simulink model "pasp_16ip_16ch"  (Simulink 6.2)
settings: Solver=ode45  StartTime=0.0  StopTime=30000  RelTol=1e-3
undefined symbols (not defined in the file or in its folder): iBOB
libraries: xbsIndex_r3 x1479, casper_library x149, xps_library x58
(part 3 of 11)

== system pasp_16ip_16ch/pasp/reorder ==
  sync : Inport  Port=1  LatchInput=off
  en : Inport  Port=2  LatchInput=off
  din0 : Inport  Port=3  LatchInput=off
  din1 : Inport  Port=4  LatchInput=off
  Counter : xbsIndex_r3/Counter  cnt_type=Count Limited  n_bits=6  bin_pt=0  arith_type=Unsigned  start_count=0  cnt_to=63  cnt_by_val=1  operation=Up  explicit_period=off  period=1  load_pin=off  rst=on  en=on  dbl_ovrd=off  show_param=off  use_rpm=on  gen_core=off
      settings: xl_area=[0, 0, 0, 0, 0, 0, 0]
  Mux : xbsIndex_r3/Mux  inputs=4  precision=Full  arith_type="Signed  (2's comp)"  n_bits=8  bin_pt=2  quantization=Truncate  overflow=Wrap  latency=1  explicit_period=off  period=1  en=off  dbl_ovrd=off  show_param=off  mux_type=off  use_rpm=off  gen_core=off
      settings: xl_area=[0, 0, 0, 0, 0, 0, 0]
  Slice1 : xbsIndex_r3/Slice  mode=Upper Bit Location + Width  nbits=2  bit1=0  base1=MSB of Input  bit0=0  base0=LSB of Input  boolean_output=off  explicit_period=off  period=1  dbl_ovrd=off
  Slice2 : xbsIndex_r3/Slice  mode=Lower Bit Location + Width  nbits=4  bit1=0  base1=MSB of Input  bit0=0  base0=LSB of Input  boolean_output=off  explicit_period=off  period=1  dbl_ovrd=off
  bram0 : xbsIndex_r3/Single Port RAM  depth=16  initVector=sin(pi*(0:15)/16)  write_mode=Read Before Write  latency=2  init_zero=on  explicit_period=off  period=1  rst=off  init_reg=0  en=off  dbl_ovrd=off  show_param=off  distributed_mem=off  use_rpm=off  gen_core=off
      settings: xl_area=[0, 0, 0, 0, 0, 0, 0]
  bram1 : xbsIndex_r3/Single Port RAM  depth=16  initVector=sin(pi*(0:15)/16)  write_mode=Read Before Write  latency=2  init_zero=on  explicit_period=off  period=1  rst=off  init_reg=0  en=off  dbl_ovrd=off  show_param=off  distributed_mem=off  use_rpm=off  gen_core=off
      settings: xl_area=[0, 0, 0, 0, 0, 0, 0]
  delay_d0 : xbsIndex_r3/Delay  latency=3  reg_retiming=off  explicit_period=off  period=1  en=off  accept_only_valid=off  init_zero=on  dbl_ovrd=off  show_param=off
      settings: xl_area=[0, 0, 0, 0, 0, 0, 0]
  delay_din0 : xbsIndex_r3/Delay  latency=4  reg_retiming=off  explicit_period=off  period=1  en=off  accept_only_valid=off  init_zero=on  dbl_ovrd=off  show_param=off
      settings: xl_area=[0, 0, 0, 0, 0, 0, 0]
  delay_din1 : xbsIndex_r3/Delay  latency=4  reg_retiming=off  explicit_period=off  period=1  en=off  accept_only_valid=off  init_zero=on  dbl_ovrd=off  show_param=off
      settings: xl_area=[0, 0, 0, 0, 0, 0, 0]
  delay_map1 : xbsIndex_r3/Delay  latency=2*map_latency  reg_retiming=off  explicit_period=off  period=1  en=off  accept_only_valid=off  init_zero=on  dbl_ovrd=off  show_param=off
      settings: xl_area=[0, 0, 0, 0, 0, 0, 0]
  delay_map2 : xbsIndex_r3/Delay  latency=1*map_latency  reg_retiming=off  explicit_period=off  period=1  en=off  accept_only_valid=off  init_zero=on  dbl_ovrd=off  show_param=off
      settings: xl_area=[0, 0, 0, 0, 0, 0, 0]
  delay_map3 : xbsIndex_r3/Delay  latency=0*map_latency  reg_retiming=off  explicit_period=off  period=1  en=off  accept_only_valid=off  init_zero=on  dbl_ovrd=off  show_param=off
      settings: xl_area=[0, 0, 0, 0, 0, 0, 0]
  delay_sel : xbsIndex_r3/Delay  latency=3  reg_retiming=off  explicit_period=off  period=1  en=off  accept_only_valid=off  init_zero=on  dbl_ovrd=off  show_param=off
      settings: xl_area=[0, 0, 0, 0, 0, 0, 0]
  delay_valid : xbsIndex_r3/Delay  latency=3  reg_retiming=off  explicit_period=off  period=1  en=off  accept_only_valid=off  init_zero=on  dbl_ovrd=off  show_param=off
      settings: xl_area=[0, 0, 0, 0, 0, 0, 0]
  delay_we : xbsIndex_r3/Delay  latency=3  reg_retiming=off  explicit_period=off  period=1  en=off  accept_only_valid=off  init_zero=on  dbl_ovrd=off  show_param=off
      settings: xl_area=[0, 0, 0, 0, 0, 0, 0]
  map1 : xbsIndex_r3/ROM  depth=16  initVector=[0 8 1 9 2 10 3 11 4 12 5 13 6 14 7 15]  arith_type=Unsigned  n_bits=4  bin_pt=0  latency=1  init_zero=on  explicit_period=off  period=1  rst=off  init_reg=0  en=off  dbl_ovrd=off  show_param=off  distributed_mem=on  use_rpm=off  gen_core=off
      settings: xl_area=[0, 0, 0, 0, 0, 0, 0]
  map2 : xbsIndex_r3/ROM  depth=16  initVector=[0 8 1 9 2 10 3 11 4 12 5 13 6 14 7 15]  arith_type=Unsigned  n_bits=4  bin_pt=0  latency=1  init_zero=on  explicit_period=off  period=1  rst=off  init_reg=0  en=off  dbl_ovrd=off  show_param=off  distributed_mem=on  use_rpm=off  gen_core=off
      settings: xl_area=[0, 0, 0, 0, 0, 0, 0]
  map3 : xbsIndex_r3/ROM  depth=16  initVector=[0 8 1 9 2 10 3 11 4 12 5 13 6 14 7 15]  arith_type=Unsigned  n_bits=4  bin_pt=0  latency=1  init_zero=on  explicit_period=off  period=1  rst=off  init_reg=0  en=off  dbl_ovrd=off  show_param=off  distributed_mem=on  use_rpm=off  gen_core=off
      settings: xl_area=[0, 0, 0, 0, 0, 0, 0]
  post_sync_delay : xbsIndex_r3/Delay  latency=3  reg_retiming=off  explicit_period=off  period=1  en=off  accept_only_valid=off  init_zero=on  dbl_ovrd=off  show_param=off
      settings: xl_area=[0, 0, 0, 0, 0, 0, 0]
  pre_sync_delay : xbsIndex_r3/Delay  latency=3  reg_retiming=off  explicit_period=off  period=1  en=off  accept_only_valid=off  init_zero=on  dbl_ovrd=off  show_param=off
      settings: xl_area=[0, 0, 0, 0, 0, 0, 0]
  sync_delay_en : casper_library/Delays/sync_delay_en  DelayLen=16
      link override Constant: equ=P=C
      link override Constant1: equ=P=C
      link override Constant2: equ=P=C
      link override Constant3: equ=P=C
  sync_out : Outport
  valid : Outport  Port=2
  dout0 : Outport  Port=3
  dout1 : Outport  Port=4
  wires:
  sync/1 -> Counter/1, pre_sync_delay/1
  en/1 -> Counter/2, sync_delay_en/2, delay_we/1
  Counter/1 -> Slice1/1, Slice2/1
  Slice1/1 -> delay_sel/1
  delay_sel/1 -> Mux/1
  Slice2/1 -> delay_d0/1, map1/1
  delay_d0/1 -> Mux/2
  pre_sync_delay/1 -> sync_delay_en/1
  sync_delay_en/1 -> post_sync_delay/1
  post_sync_delay/1 -> sync_out/1
  delay_we/1 -> delay_valid/1, bram0/3, bram1/3
  delay_valid/1 -> valid/1
  Mux/1 -> bram0/1, bram1/1
  din0/1 -> delay_din0/1
  delay_din0/1 -> bram0/2
  bram0/1 -> dout0/1
  din1/1 -> delay_din1/1
  delay_din1/1 -> bram1/2
  bram1/1 -> dout1/1
  map1/1 -> delay_map1/1, map2/1
  delay_map1/1 -> Mux/3
  map2/1 -> delay_map2/1, map3/1
  delay_map2/1 -> Mux/4
  map3/1 -> delay_map3/1
  delay_map3/1 -> Mux/5

== system pasp_16ip_16ch/pasp/scale1 ==
  note: Unsigned, 18-bits, b.p. at 12
  note: Output complex signed R/I 18-bits, b.p. at 17
  note: Input complex signed R/I 18-bits, b.p. at 17
  coeff : Inport  Orientation=down  Port=1  LatchInput=off
  data_in : Inport  Port=2  LatchInput=off
  c_to_ri : casper_library/Misc/c_to_ri  n_bits=18  bin_pt=17
      settings: AttributesFormatString=18_17 r/i
  mult_coeff_fft_imag : xbsIndex_r3/Mult  precision=User Defined  arith_type="Signed  (2's comp)"  n_bits=18  bin_pt=17  quantization=Truncate  overflow=Saturate  latency=6  explicit_period=off  period=1  en=off  dbl_ovrd=off  show_param=on  mult_type=Parallel  oversample=2  use_embedded=on  pipeline=on  use_rpm=on  placement_style=Rectangular Shape  gen_core=off
      settings: xl_area=[0, 0, 0, 0, 0, 0, 0]
  mult_coeff_fft_real : xbsIndex_r3/Mult  precision=User Defined  arith_type="Signed  (2's comp)"  n_bits=18  bin_pt=17  quantization=Truncate  overflow=Saturate  latency=6  explicit_period=off  period=1  en=off  dbl_ovrd=off  show_param=on  mult_type=Parallel  oversample=2  use_embedded=on  pipeline=on  use_rpm=on  placement_style=Rectangular Shape  gen_core=off
      settings: xl_area=[0, 0, 0, 0, 0, 0, 0]
  ri_to_c : casper_library/Misc/ri_to_c
  data_out : Outport
  wires:
  c_to_ri/1 -> mult_coeff_fft_real/2
  c_to_ri/2 -> mult_coeff_fft_imag/2
  mult_coeff_fft_real/1 -> ri_to_c/1
  mult_coeff_fft_imag/1 -> ri_to_c/2
  coeff/1 -> mult_coeff_fft_real/1, mult_coeff_fft_imag/1
  ri_to_c/1 -> data_out/1
  data_in/1 -> c_to_ri/1

== system pasp_16ip_16ch/pasp/scale2 ==
  note: Input complex signed R/I 18-bits, b.p. at 17
  note: Output complex signed R/I 18-bits, b.p. at 17
  note: Unsigned, 18-bits, b.p. at 12
  coeff : Inport  Orientation=down  Port=1  LatchInput=off
  data_in : Inport  Port=2  LatchInput=off
  c_to_ri : casper_library/Misc/c_to_ri  n_bits=18  bin_pt=17
      settings: AttributesFormatString=18_17 r/i
  mult_coeff_fft_imag : xbsIndex_r3/Mult  precision=User Defined  arith_type="Signed  (2's comp)"  n_bits=18  bin_pt=17  quantization=Truncate  overflow=Saturate  latency=6  explicit_period=off  period=1  en=off  dbl_ovrd=off  show_param=on  mult_type=Parallel  oversample=2  use_embedded=on  pipeline=on  use_rpm=on  placement_style=Rectangular Shape  gen_core=off
      settings: xl_area=[0, 0, 0, 0, 0, 0, 0]
  mult_coeff_fft_real : xbsIndex_r3/Mult  precision=User Defined  arith_type="Signed  (2's comp)"  n_bits=18  bin_pt=17  quantization=Truncate  overflow=Saturate  latency=6  explicit_period=off  period=1  en=off  dbl_ovrd=off  show_param=on  mult_type=Parallel  oversample=2  use_embedded=on  pipeline=on  use_rpm=on  placement_style=Rectangular Shape  gen_core=off
      settings: xl_area=[0, 0, 0, 0, 0, 0, 0]
  ri_to_c : casper_library/Misc/ri_to_c
  data_out : Outport
  wires:
  data_in/1 -> c_to_ri/1
  ri_to_c/1 -> data_out/1
  coeff/1 -> mult_coeff_fft_imag/1, mult_coeff_fft_real/1
  mult_coeff_fft_imag/1 -> ri_to_c/2
  mult_coeff_fft_real/1 -> ri_to_c/1
  c_to_ri/2 -> mult_coeff_fft_imag/2
  c_to_ri/1 -> mult_coeff_fft_real/2

== system pasp_16ip_16ch/pasp/scale3 ==
  note: Unsigned, 18-bits, b.p. at 12
  note: Output complex signed R/I 18-bits, b.p. at 17
  note: Input complex signed R/I 18-bits, b.p. at 17
  coeff : Inport  Orientation=down  Port=1  LatchInput=off
  data_in : Inport  Port=2  LatchInput=off
  c_to_ri : casper_library/Misc/c_to_ri  n_bits=18  bin_pt=17
      settings: AttributesFormatString=18_17 r/i
  mult_coeff_fft_imag : xbsIndex_r3/Mult  precision=User Defined  arith_type="Signed  (2's comp)"  n_bits=18  bin_pt=17  quantization=Truncate  overflow=Saturate  latency=6  explicit_period=off  period=1  en=off  dbl_ovrd=off  show_param=on  mult_type=Parallel  oversample=2  use_embedded=on  pipeline=on  use_rpm=on  placement_style=Rectangular Shape  gen_core=off
      settings: xl_area=[0, 0, 0, 0, 0, 0, 0]
  mult_coeff_fft_real : xbsIndex_r3/Mult  precision=User Defined  arith_type="Signed  (2's comp)"  n_bits=18  bin_pt=17  quantization=Truncate  overflow=Saturate  latency=6  explicit_period=off  period=1  en=off  dbl_ovrd=off  show_param=on  mult_type=Parallel  oversample=2  use_embedded=on  pipeline=on  use_rpm=on  placement_style=Rectangular Shape  gen_core=off
      settings: xl_area=[0, 0, 0, 0, 0, 0, 0]
  ri_to_c : casper_library/Misc/ri_to_c
  data_out : Outport
  wires:
  c_to_ri/1 -> mult_coeff_fft_real/2
  c_to_ri/2 -> mult_coeff_fft_imag/2
  mult_coeff_fft_real/1 -> ri_to_c/1
  mult_coeff_fft_imag/1 -> ri_to_c/2
  coeff/1 -> mult_coeff_fft_real/1, mult_coeff_fft_imag/1
  ri_to_c/1 -> data_out/1
  data_in/1 -> c_to_ri/1

== system pasp_16ip_16ch/pasp/scale4 ==
  note: Input complex signed R/I 18-bits, b.p. at 17
  note: Output complex signed R/I 18-bits, b.p. at 17
  note: Unsigned, 18-bits, b.p. at 12
  coeff : Inport  Orientation=down  Port=1  LatchInput=off
  data_in : Inport  Port=2  LatchInput=off
  c_to_ri : casper_library/Misc/c_to_ri  n_bits=18  bin_pt=17
      settings: AttributesFormatString=18_17 r/i
  mult_coeff_fft_imag : xbsIndex_r3/Mult  precision=User Defined  arith_type="Signed  (2's comp)"  n_bits=18  bin_pt=17  quantization=Truncate  overflow=Saturate  latency=6  explicit_period=off  period=1  en=off  dbl_ovrd=off  show_param=on  mult_type=Parallel  oversample=2  use_embedded=on  pipeline=on  use_rpm=on  placement_style=Rectangular Shape  gen_core=off
      settings: xl_area=[0, 0, 0, 0, 0, 0, 0]
  mult_coeff_fft_real : xbsIndex_r3/Mult  precision=User Defined  arith_type="Signed  (2's comp)"  n_bits=18  bin_pt=17  quantization=Truncate  overflow=Saturate  latency=6  explicit_period=off  period=1  en=off  dbl_ovrd=off  show_param=on  mult_type=Parallel  oversample=2  use_embedded=on  pipeline=on  use_rpm=on  placement_style=Rectangular Shape  gen_core=off
      settings: xl_area=[0, 0, 0, 0, 0, 0, 0]
  ri_to_c : casper_library/Misc/ri_to_c
  data_out : Outport
  wires:
  data_in/1 -> c_to_ri/1
  ri_to_c/1 -> data_out/1
  coeff/1 -> mult_coeff_fft_imag/1, mult_coeff_fft_real/1
  mult_coeff_fft_imag/1 -> ri_to_c/2
  mult_coeff_fft_real/1 -> ri_to_c/1
  c_to_ri/2 -> mult_coeff_fft_imag/2
  c_to_ri/1 -> mult_coeff_fft_real/2

== system pasp_16ip_16ch/pasp/scope_output1 ==
  rst : Inport  Port=1  LatchInput=off
  en : Inport  Port=2  LatchInput=off
  data_in : Inport  Port=3  LatchInput=off
  bram : xps_library/Shared BRAM  Tag=xps:bram  arith_type="Signed  (2's comp)"  addr_width=11  data_width=32  data_bin_pt=17  init_vals=[1:2^11]  sample_rate=1
  freeze_cntr : casper_library/Misc/freeze_cntr  CounterBits=11
  wires:
  freeze_cntr/1 -> bram/1
  freeze_cntr/2 -> bram/3
  en/1 -> freeze_cntr/1
  data_in/1 -> bram/2
  rst/1 -> freeze_cntr/2

== system pasp_16ip_16ch/pasp/scope_output2 ==
  rst : Inport  Port=1  LatchInput=off
  en : Inport  Port=2  LatchInput=off
  data_in : Inport  Port=3  LatchInput=off
  bram : xps_library/Shared BRAM  Tag=xps:bram  arith_type="Signed  (2's comp)"  addr_width=11  data_width=32  data_bin_pt=17  init_vals=[1:2^11]  sample_rate=1
  freeze_cntr : casper_library/Misc/freeze_cntr  CounterBits=11
  wires:
  freeze_cntr/1 -> bram/1
  freeze_cntr/2 -> bram/3
  en/1 -> freeze_cntr/1
  data_in/1 -> bram/2
  rst/1 -> freeze_cntr/2

== system pasp_16ip_16ch/pasp/scope_output3 ==
  rst : Inport  Port=1  LatchInput=off
  en : Inport  Port=2  LatchInput=off
  data_in : Inport  Port=3  LatchInput=off
  bram : xps_library/Shared BRAM  Tag=xps:bram  arith_type="Signed  (2's comp)"  addr_width=11  data_width=32  data_bin_pt=17  init_vals=[1:2^11]  sample_rate=1
  freeze_cntr : casper_library/Misc/freeze_cntr  CounterBits=11
  wires:
  rst/1 -> freeze_cntr/2
  data_in/1 -> bram/2
  en/1 -> freeze_cntr/1
  freeze_cntr/2 -> bram/3
  freeze_cntr/1 -> bram/1

== system pasp_16ip_16ch/pasp/scope_output4 ==
  rst : Inport  Port=1  LatchInput=off
  en : Inport  Port=2  LatchInput=off
  data_in : Inport  Port=3  LatchInput=off
  bram : xps_library/Shared BRAM  Tag=xps:bram  arith_type="Signed  (2's comp)"  addr_width=11  data_width=32  data_bin_pt=17  init_vals=[1:2^11]  sample_rate=1
  freeze_cntr : casper_library/Misc/freeze_cntr  CounterBits=11
  wires:
  freeze_cntr/1 -> bram/1
  freeze_cntr/2 -> bram/3
  en/1 -> freeze_cntr/1
  data_in/1 -> bram/2
  rst/1 -> freeze_cntr/2

== system pasp_16ip_16ch/pasp/scope_output5 ==
  rst : Inport  Port=1  LatchInput=off
  en : Inport  Port=2  LatchInput=off
  data_in : Inport  Port=3  LatchInput=off
  bram : xps_library/Shared BRAM  Tag=xps:bram  arith_type="Signed  (2's comp)"  addr_width=11  data_width=32  data_bin_pt=17  init_vals=[1:2^11]  sample_rate=1
  freeze_cntr : casper_library/Misc/freeze_cntr  CounterBits=11
  wires:
  freeze_cntr/1 -> bram/1
  freeze_cntr/2 -> bram/3
  en/1 -> freeze_cntr/1
  data_in/1 -> bram/2
  rst/1 -> freeze_cntr/2

== system pasp_16ip_16ch/pasp/scope_output6 ==
  rst : Inport  Port=1  LatchInput=off
  en : Inport  Port=2  LatchInput=off
  data_in : Inport  Port=3  LatchInput=off
  bram : xps_library/Shared BRAM  Tag=xps:bram  arith_type="Signed  (2's comp)"  addr_width=11  data_width=32  data_bin_pt=17  init_vals=[1:2^11]  sample_rate=1
  freeze_cntr : casper_library/Misc/freeze_cntr  CounterBits=11
  wires:
  freeze_cntr/1 -> bram/1
  freeze_cntr/2 -> bram/3
  en/1 -> freeze_cntr/1
  data_in/1 -> bram/2
  rst/1 -> freeze_cntr/2

== system pasp_16ip_16ch/pasp/scope_output7 ==
  rst : Inport  Port=1  LatchInput=off
  en : Inport  Port=2  LatchInput=off
  data_in : Inport  Port=3  LatchInput=off
  bram : xps_library/Shared BRAM  Tag=xps:bram  arith_type="Signed  (2's comp)"  addr_width=11  data_width=32  data_bin_pt=17  init_vals=[1:2^11]  sample_rate=1
  freeze_cntr : casper_library/Misc/freeze_cntr  CounterBits=11
  wires:
  rst/1 -> freeze_cntr/2
  data_in/1 -> bram/2
  en/1 -> freeze_cntr/1
  freeze_cntr/2 -> bram/3
  freeze_cntr/1 -> bram/1

== system pasp_16ip_16ch/pasp/scope_output8 ==
  rst : Inport  Port=1  LatchInput=off
  en : Inport  Port=2  LatchInput=off
  data_in : Inport  Port=3  LatchInput=off
  bram : xps_library/Shared BRAM  Tag=xps:bram  arith_type="Signed  (2's comp)"  addr_width=11  data_width=32  data_bin_pt=17  init_vals=[1:2^11]  sample_rate=1
  freeze_cntr : casper_library/Misc/freeze_cntr  CounterBits=11
  wires:
  freeze_cntr/1 -> bram/1
  freeze_cntr/2 -> bram/3
  en/1 -> freeze_cntr/1
  data_in/1 -> bram/2
  rst/1 -> freeze_cntr/2

== system pasp_16ip_16ch/pasp/sync_generator ==
  period : Inport  Port=1  LatchInput=off
  reset : Inport  Port=2  LatchInput=off
  Convert : xbsIndex_r3/Convert  arith_type=Boolean  n_bits=8  bin_pt=6  quantization=Truncate  overflow=Wrap  latency=1  explicit_period=off  period=1  dbl_ovrd=off  show_param=off  inserted_by_tool=off  pipeline=off
      settings: xl_area=[0, 0, 0, 0, 0, 0, 0]
  Counter : xbsIndex_r3/Counter  cnt_type=Free Running  n_bits=32  bin_pt=0  arith_type=Unsigned  start_count=1  cnt_to=Inf  cnt_by_val=1  operation=Up  explicit_period=on  period=1  load_pin=off  rst=on  en=off  dbl_ovrd=off  show_param=off  use_rpm=on  gen_core=off
      settings: xl_area=[0, 0, 0, 0, 0, 0, 0]
  Logical : xbsIndex_r3/Logical  logical_function=OR  inputs=2  precision=Full  arith_type=Unsigned  n_bits=8  bin_pt=2  align_bp=on  latency=0  explicit_period=off  period=1  en=off  dbl_ovrd=off  show_param=off
      settings: xl_area=[0, 0, 0, 0, 0, 0, 0]
  Relational : xbsIndex_r3/Relational  mode=a>=b  latency=1  explicit_period=off  period=1  en=off  dbl_ovrd=off  show_param=off
      settings: xl_area=[0, 0, 0, 0, 0, 0, 0]
  cns : xbsIndex_r3/Constant  const=4  equ=P=C  arith_type=Unsigned  n_bits=3  bin_pt=0  opselect=C  inp2=PCIN>>17  opr=+  inp1=P  carry=CIN  iostate=0  explicit_period=off  period=1  dbl_ovrd=off
  period_sub : xbsIndex_r3/AddSub  mode=Subtraction  precision=User Defined  arith_type=Unsigned  n_bits=32  bin_pt=0  quantization=Truncate  overflow=Wrap  latency=0  explicit_period=off  period=1  use_carryin=off  use_carryout=off  en=off  dbl_ovrd=off  show_param=off  use_core=on  pipeline=off  use_rpm=on  gen_core=off
      settings: xl_area=[0, 0, 0, 0, 0, 0, 0]
  posedge : casper_library/Misc/posedge  Tag=Rising Edge Detector
  sync : Outport
  wires:
  Counter/1 -> Relational/1
  Relational/1 -> Convert/1
  Convert/1 -> Logical/2
  Logical/1 -> Counter/1, posedge/1
  reset/1 -> Logical/1
  period/1 -> period_sub/1
  period_sub/1 -> Relational/2
  cns/1 -> period_sub/2
  posedge/1 -> sync/1

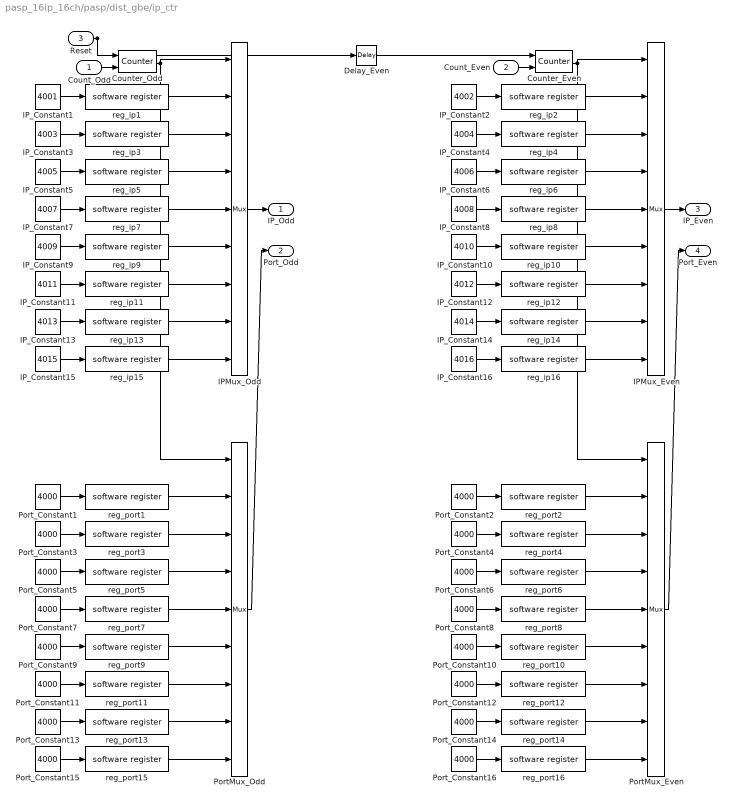
== system pasp_16ip_16ch/pasp/dist_gbe/ip_ctr ==
  Count_Odd : Inport  Port=1  LatchInput=off
  Count_Even : Inport  Port=2  LatchInput=off
  Reset : Inport  Port=3  LatchInput=off
  Counter_Even : xbsIndex_r3/Counter  cnt_type=Free Running  n_bits=3  bin_pt=0  arith_type=Unsigned  start_count=0  cnt_to=Inf  cnt_by_val=1  operation=Up  explicit_period=off  period=1  load_pin=off  rst=on  en=on  dbl_ovrd=off  show_param=off  use_rpm=on  gen_core=off
      settings: xl_area=[0, 0, 0, 0, 0, 0, 0]
  Counter_Odd : xbsIndex_r3/Counter  cnt_type=Free Running  n_bits=3  bin_pt=0  arith_type=Unsigned  start_count=0  cnt_to=Inf  cnt_by_val=1  operation=Up  explicit_period=off  period=1  load_pin=off  rst=on  en=on  dbl_ovrd=off  show_param=off  use_rpm=on  gen_core=off
      settings: xl_area=[0, 0, 0, 0, 0, 0, 0]
  Delay_Even : xbsIndex_r3/Delay  latency=4  reg_retiming=off  explicit_period=off  period=1  en=off  accept_only_valid=off  init_zero=on  dbl_ovrd=off  show_param=off
      settings: xl_area=[0, 0, 0, 0, 0, 0, 0]
  IPMux_Even : xbsIndex_r3/Mux  inputs=8  precision=Full  arith_type="Signed  (2's comp)"  n_bits=8  bin_pt=2  quantization=Truncate  overflow=Wrap  latency=3  explicit_period=off  period=1  en=off  dbl_ovrd=off  show_param=off  mux_type=off  use_rpm=off  gen_core=off
      settings: xl_area=[0, 0, 0, 0, 0, 0, 0]
  IPMux_Odd : xbsIndex_r3/Mux  inputs=8  precision=Full  arith_type="Signed  (2's comp)"  n_bits=8  bin_pt=2  quantization=Truncate  overflow=Wrap  latency=3  explicit_period=off  period=1  en=off  dbl_ovrd=off  show_param=off  mux_type=off  use_rpm=off  gen_core=off
      settings: xl_area=[0, 0, 0, 0, 0, 0, 0]
  IP_Constant1 : Constant  Value=4001
  IP_Constant10 : Constant  Value=4010
  IP_Constant11 : Constant  Value=4011
  IP_Constant12 : Constant  Value=4012
  IP_Constant13 : Constant  Value=4013
  IP_Constant14 : Constant  Value=4014
  IP_Constant15 : Constant  Value=4015
  IP_Constant16 : Constant  Value=4016
  IP_Constant2 : Constant  Value=4002
  IP_Constant3 : Constant  Value=4003
  IP_Constant4 : Constant  Value=4004
  IP_Constant5 : Constant  Value=4005
  IP_Constant6 : Constant  Value=4006
  IP_Constant7 : Constant  Value=4007
  IP_Constant8 : Constant  Value=4008
  IP_Constant9 : Constant  Value=4009
  PortMux_Even : xbsIndex_r3/Mux  inputs=8  precision=Full  arith_type="Signed  (2's comp)"  n_bits=8  bin_pt=2  quantization=Truncate  overflow=Wrap  latency=3  explicit_period=off  period=1  en=off  dbl_ovrd=off  show_param=off  mux_type=off  use_rpm=off  gen_core=off
      settings: xl_area=[0, 0, 0, 0, 0, 0, 0]
  PortMux_Odd : xbsIndex_r3/Mux  inputs=8  precision=Full  arith_type="Signed  (2's comp)"  n_bits=8  bin_pt=2  quantization=Truncate  overflow=Wrap  latency=3  explicit_period=off  period=1  en=off  dbl_ovrd=off  show_param=off  mux_type=off  use_rpm=off  gen_core=off
      settings: xl_area=[0, 0, 0, 0, 0, 0, 0]
  Port_Constant{1..16} (16 alike) : Constant  Value=4000
  reg_ip1 : xps_library/software register  Tag=xps:sw_reg  io_dir=From Processor  arith_type=Unsigned  bitwidth=32  bin_pt=0  sample_period=1  gw_name=pasp_16ip_16ch_pasp_dist_gbe_ip_ctr_reg_ip1_user_data_out
  reg_ip10 : xps_library/software register  Tag=xps:sw_reg  io_dir=From Processor  arith_type=Unsigned  bitwidth=32  bin_pt=0  sample_period=1  gw_name=pasp_16ip_16ch_pasp_dist_gbe_ip_ctr_reg_ip10_user_data_out
  reg_ip11 : xps_library/software register  Tag=xps:sw_reg  io_dir=From Processor  arith_type=Unsigned  bitwidth=32  bin_pt=0  sample_period=1  gw_name=pasp_16ip_16ch_pasp_dist_gbe_ip_ctr_reg_ip11_user_data_out
  reg_ip12 : xps_library/software register  Tag=xps:sw_reg  io_dir=From Processor  arith_type=Unsigned  bitwidth=32  bin_pt=0  sample_period=1  gw_name=pasp_16ip_16ch_pasp_dist_gbe_ip_ctr_reg_ip12_user_data_out
  reg_ip13 : xps_library/software register  Tag=xps:sw_reg  io_dir=From Processor  arith_type=Unsigned  bitwidth=32  bin_pt=0  sample_period=1  gw_name=pasp_16ip_16ch_pasp_dist_gbe_ip_ctr_reg_ip13_user_data_out
  reg_ip14 : xps_library/software register  Tag=xps:sw_reg  io_dir=From Processor  arith_type=Unsigned  bitwidth=32  bin_pt=0  sample_period=1  gw_name=pasp_16ip_16ch_pasp_dist_gbe_ip_ctr_reg_ip14_user_data_out
  reg_ip15 : xps_library/software register  Tag=xps:sw_reg  io_dir=From Processor  arith_type=Unsigned  bitwidth=32  bin_pt=0  sample_period=1  gw_name=pasp_16ip_16ch_pasp_dist_gbe_ip_ctr_reg_ip15_user_data_out
  reg_ip16 : xps_library/software register  Tag=xps:sw_reg  io_dir=From Processor  arith_type=Unsigned  bitwidth=32  bin_pt=0  sample_period=1  gw_name=pasp_16ip_16ch_pasp_dist_gbe_ip_ctr_reg_ip16_user_data_out
  reg_ip2 : xps_library/software register  Tag=xps:sw_reg  io_dir=From Processor  arith_type=Unsigned  bitwidth=32  bin_pt=0  sample_period=1  gw_name=pasp_16ip_16ch_pasp_dist_gbe_ip_ctr_reg_ip2_user_data_out
  reg_ip3 : xps_library/software register  Tag=xps:sw_reg  io_dir=From Processor  arith_type=Unsigned  bitwidth=32  bin_pt=0  sample_period=1  gw_name=pasp_16ip_16ch_pasp_dist_gbe_ip_ctr_reg_ip3_user_data_out
  reg_ip4 : xps_library/software register  Tag=xps:sw_reg  io_dir=From Processor  arith_type=Unsigned  bitwidth=32  bin_pt=0  sample_period=1  gw_name=pasp_16ip_16ch_pasp_dist_gbe_ip_ctr_reg_ip4_user_data_out
  reg_ip5 : xps_library/software register  Tag=xps:sw_reg  io_dir=From Processor  arith_type=Unsigned  bitwidth=32  bin_pt=0  sample_period=1  gw_name=pasp_16ip_16ch_pasp_dist_gbe_ip_ctr_reg_ip5_user_data_out
  reg_ip6 : xps_library/software register  Tag=xps:sw_reg  io_dir=From Processor  arith_type=Unsigned  bitwidth=32  bin_pt=0  sample_period=1  gw_name=pasp_16ip_16ch_pasp_dist_gbe_ip_ctr_reg_ip6_user_data_out
  reg_ip7 : xps_library/software register  Tag=xps:sw_reg  io_dir=From Processor  arith_type=Unsigned  bitwidth=32  bin_pt=0  sample_period=1  gw_name=pasp_16ip_16ch_pasp_dist_gbe_ip_ctr_reg_ip7_user_data_out
  reg_ip8 : xps_library/software register  Tag=xps:sw_reg  io_dir=From Processor  arith_type=Unsigned  bitwidth=32  bin_pt=0  sample_period=1  gw_name=pasp_16ip_16ch_pasp_dist_gbe_ip_ctr_reg_ip8_user_data_out
  reg_ip9 : xps_library/software register  Tag=xps:sw_reg  io_dir=From Processor  arith_type=Unsigned  bitwidth=32  bin_pt=0  sample_period=1  gw_name=pasp_16ip_16ch_pasp_dist_gbe_ip_ctr_reg_ip9_user_data_out
  reg_port1 : xps_library/software register  Tag=xps:sw_reg  io_dir=From Processor  arith_type=Unsigned  bitwidth=32  bin_pt=0  sample_period=1  gw_name=pasp_16ip_16ch_pasp_dist_gbe_ip_ctr_reg_port1_user_data_out
  reg_port10 : xps_library/software register  Tag=xps:sw_reg  io_dir=From Processor  arith_type=Unsigned  bitwidth=32  bin_pt=0  sample_period=1  gw_name=pasp_16ip_16ch_pasp_dist_gbe_ip_ctr_reg_port10_user_data_out
  reg_port11 : xps_library/software register  Tag=xps:sw_reg  io_dir=From Processor  arith_type=Unsigned  bitwidth=32  bin_pt=0  sample_period=1  gw_name=pasp_16ip_16ch_pasp_dist_gbe_ip_ctr_reg_port11_user_data_out
  reg_port12 : xps_library/software register  Tag=xps:sw_reg  io_dir=From Processor  arith_type=Unsigned  bitwidth=32  bin_pt=0  sample_period=1  gw_name=pasp_16ip_16ch_pasp_dist_gbe_ip_ctr_reg_port12_user_data_out
  reg_port13 : xps_library/software register  Tag=xps:sw_reg  io_dir=From Processor  arith_type=Unsigned  bitwidth=32  bin_pt=0  sample_period=1  gw_name=pasp_16ip_16ch_pasp_dist_gbe_ip_ctr_reg_port13_user_data_out
  reg_port14 : xps_library/software register  Tag=xps:sw_reg  io_dir=From Processor  arith_type=Unsigned  bitwidth=32  bin_pt=0  sample_period=1  gw_name=pasp_16ip_16ch_pasp_dist_gbe_ip_ctr_reg_port14_user_data_out
  reg_port15 : xps_library/software register  Tag=xps:sw_reg  io_dir=From Processor  arith_type=Unsigned  bitwidth=32  bin_pt=0  sample_period=1  gw_name=pasp_16ip_16ch_pasp_dist_gbe_ip_ctr_reg_port15_user_data_out
  reg_port16 : xps_library/software register  Tag=xps:sw_reg  io_dir=From Processor  arith_type=Unsigned  bitwidth=32  bin_pt=0  sample_period=1  gw_name=pasp_16ip_16ch_pasp_dist_gbe_ip_ctr_reg_port16_user_data_out
  reg_port2 : xps_library/software register  Tag=xps:sw_reg  io_dir=From Processor  arith_type=Unsigned  bitwidth=32  bin_pt=0  sample_period=1  gw_name=pasp_16ip_16ch_pasp_dist_gbe_ip_ctr_reg_port2_user_data_out
  reg_port3 : xps_library/software register  Tag=xps:sw_reg  io_dir=From Processor  arith_type=Unsigned  bitwidth=32  bin_pt=0  sample_period=1  gw_name=pasp_16ip_16ch_pasp_dist_gbe_ip_ctr_reg_port3_user_data_out
  reg_port4 : xps_library/software register  Tag=xps:sw_reg  io_dir=From Processor  arith_type=Unsigned  bitwidth=32  bin_pt=0  sample_period=1  gw_name=pasp_16ip_16ch_pasp_dist_gbe_ip_ctr_reg_port4_user_data_out
  reg_port5 : xps_library/software register  Tag=xps:sw_reg  io_dir=From Processor  arith_type=Unsigned  bitwidth=32  bin_pt=0  sample_period=1  gw_name=pasp_16ip_16ch_pasp_dist_gbe_ip_ctr_reg_port5_user_data_out
  reg_port6 : xps_library/software register  Tag=xps:sw_reg  io_dir=From Processor  arith_type=Unsigned  bitwidth=32  bin_pt=0  sample_period=1  gw_name=pasp_16ip_16ch_pasp_dist_gbe_ip_ctr_reg_port6_user_data_out
  reg_port7 : xps_library/software register  Tag=xps:sw_reg  io_dir=From Processor  arith_type=Unsigned  bitwidth=32  bin_pt=0  sample_period=1  gw_name=pasp_16ip_16ch_pasp_dist_gbe_ip_ctr_reg_port7_user_data_out
  reg_port8 : xps_library/software register  Tag=xps:sw_reg  io_dir=From Processor  arith_type=Unsigned  bitwidth=32  bin_pt=0  sample_period=1  gw_name=pasp_16ip_16ch_pasp_dist_gbe_ip_ctr_reg_port8_user_data_out
  reg_port9 : xps_library/software register  Tag=xps:sw_reg  io_dir=From Processor  arith_type=Unsigned  bitwidth=32  bin_pt=0  sample_period=1  gw_name=pasp_16ip_16ch_pasp_dist_gbe_ip_ctr_reg_port9_user_data_out
  IP_Odd : Outport
  Port_Odd : Outport  Port=2
  IP_Even : Outport  Port=3
  Port_Even : Outport  Port=4
  wires:
  Reset/1 -> Counter_Odd/1, Delay_Even/1
  Count_Odd/1 -> Counter_Odd/2
  Counter_Odd/1 -> IPMux_Odd/1, PortMux_Odd/1
  IPMux_Odd/1 -> IP_Odd/1
  PortMux_Odd/1 -> Port_Odd/1
  Delay_Even/1 -> Counter_Even/1
  Count_Even/1 -> Counter_Even/2
  Counter_Even/1 -> IPMux_Even/1, PortMux_Even/1
  IPMux_Even/1 -> IP_Even/1
  PortMux_Even/1 -> Port_Even/1
  IP_Constant1/1 -> reg_ip1/1
  reg_ip1/1 -> IPMux_Odd/2
  Port_Constant1/1 -> reg_port1/1
  reg_port1/1 -> PortMux_Odd/2
  IP_Constant3/1 -> reg_ip3/1
  reg_ip3/1 -> IPMux_Odd/3
  Port_Constant3/1 -> reg_port3/1
  reg_port3/1 -> PortMux_Odd/3
  IP_Constant5/1 -> reg_ip5/1
  reg_ip5/1 -> IPMux_Odd/4
  Port_Constant5/1 -> reg_port5/1
  reg_port5/1 -> PortMux_Odd/4
  IP_Constant7/1 -> reg_ip7/1
  reg_ip7/1 -> IPMux_Odd/5
  Port_Constant7/1 -> reg_port7/1
  reg_port7/1 -> PortMux_Odd/5
  IP_Constant9/1 -> reg_ip9/1
  reg_ip9/1 -> IPMux_Odd/6
  Port_Constant9/1 -> reg_port9/1
  reg_port9/1 -> PortMux_Odd/6
  IP_Constant11/1 -> reg_ip11/1
  reg_ip11/1 -> IPMux_Odd/7
  Port_Constant11/1 -> reg_port11/1
  reg_port11/1 -> PortMux_Odd/7
  IP_Constant13/1 -> reg_ip13/1
  reg_ip13/1 -> IPMux_Odd/8
  Port_Constant13/1 -> reg_port13/1
  reg_port13/1 -> PortMux_Odd/8
  IP_Constant15/1 -> reg_ip15/1
  reg_ip15/1 -> IPMux_Odd/9
  Port_Constant15/1 -> reg_port15/1
  reg_port15/1 -> PortMux_Odd/9
  IP_Constant2/1 -> reg_ip2/1
  reg_ip2/1 -> IPMux_Even/2
  Port_Constant2/1 -> reg_port2/1
  reg_port2/1 -> PortMux_Even/2
  IP_Constant4/1 -> reg_ip4/1
  reg_ip4/1 -> IPMux_Even/3
  Port_Constant4/1 -> reg_port4/1
  reg_port4/1 -> PortMux_Even/3
  IP_Constant6/1 -> reg_ip6/1
  reg_ip6/1 -> IPMux_Even/4
  Port_Constant6/1 -> reg_port6/1
  reg_port6/1 -> PortMux_Even/4
  IP_Constant8/1 -> reg_ip8/1
  reg_ip8/1 -> IPMux_Even/5
  Port_Constant8/1 -> reg_port8/1
  reg_port8/1 -> PortMux_Even/5
  IP_Constant10/1 -> reg_ip10/1
  reg_ip10/1 -> IPMux_Even/6
  Port_Constant10/1 -> reg_port10/1
  reg_port10/1 -> PortMux_Even/6
  IP_Constant12/1 -> reg_ip12/1
  reg_ip12/1 -> IPMux_Even/7
  Port_Constant12/1 -> reg_port12/1
  reg_port12/1 -> PortMux_Even/7
  IP_Constant14/1 -> reg_ip14/1
  reg_ip14/1 -> IPMux_Even/8
  Port_Constant14/1 -> reg_port14/1
  reg_port14/1 -> PortMux_Even/8
  IP_Constant16/1 -> reg_ip16/1
  reg_ip16/1 -> IPMux_Even/9
  Port_Constant16/1 -> reg_port16/1
  reg_port16/1 -> PortMux_Even/9

== system pasp_16ip_16ch/pasp/dist_gbe/reorder ==
  sync : Inport  Port=1  LatchInput=off
  en : Inport  Port=2  LatchInput=off
  din0 : Inport  Port=3  LatchInput=off
  Counter : xbsIndex_r3/Counter  cnt_type=Count Limited  n_bits=11  bin_pt=0  arith_type=Unsigned  start_count=0  cnt_to=2047  cnt_by_val=1  operation=Up  explicit_period=off  period=1  load_pin=off  rst=on  en=on  dbl_ovrd=off  show_param=off  use_rpm=on  gen_core=off
      settings: xl_area=[0, 0, 0, 0, 0, 0, 0]
  Slice1 : xbsIndex_r3/Slice  mode=Upper Bit Location + Width  nbits=1  bit1=0  base1=MSB of Input  bit0=0  base0=LSB of Input  boolean_output=off  explicit_period=off  period=1  dbl_ovrd=off
  Slice2 : xbsIndex_r3/Slice  mode=Lower Bit Location + Width  nbits=10  bit1=0  base1=MSB of Input  bit0=0  base0=LSB of Input  boolean_output=off  explicit_period=off  period=1  dbl_ovrd=off
  dbl_buffer0 : casper_library/Reorder/dbl_buffer  depth=1024  latency=2
  delay_d0 : xbsIndex_r3/Delay  latency=1  reg_retiming=off  explicit_period=off  period=1  en=off  accept_only_valid=off  init_zero=on  dbl_ovrd=off  show_param=off
      settings: xl_area=[0, 0, 0, 0, 0, 0, 0]
  delay_din0 : xbsIndex_r3/Delay  latency=1  reg_retiming=off  explicit_period=off  period=1  en=off  accept_only_valid=off  init_zero=on  dbl_ovrd=off  show_param=off
      settings: xl_area=[0, 0, 0, 0, 0, 0, 0]
  delay_sel : xbsIndex_r3/Delay  latency=1  reg_retiming=off  explicit_period=off  period=1  en=off  accept_only_valid=off  init_zero=on  dbl_ovrd=off  show_param=off
      settings: xl_area=[0, 0, 0, 0, 0, 0, 0]
  delay_valid : xbsIndex_r3/Delay  latency=4  reg_retiming=off  explicit_period=off  period=1  en=off  accept_only_valid=off  init_zero=on  dbl_ovrd=off  show_param=off
      settings: xl_area=[0, 0, 0, 0, 0, 0, 0]
  delay_we : xbsIndex_r3/Delay  latency=1  reg_retiming=off  explicit_period=off  period=1  en=off  accept_only_valid=off  init_zero=on  dbl_ovrd=off  show_param=off
      settings: xl_area=[0, 0, 0, 0, 0, 0, 0]
  map1 : xbsIndex_r3/ROM  depth=1024  initVector=[0 16 32 48 64 80 96 112 128 144 160 176 192 208 224 240 256 272 288 304 320 336 352 368 384 400 416 432 448 464 480 496 512 528 544 560 576 592 608 624 640 656 672 688 704 720 736 752 768 784 800 816 832 848 864 880 896 912 928 944 960 976 992 1008 1 17 33 49 65 81 97 113 129 145 161 177 193 209 225 241 257 273 289 305 321 337 353 369 385 401 417 433 449 465 481 497 513 529 545 561 577 593 609 625 641 657 673 689 705 721 737 753 769 785 801 817 833 849 865 881 897 913 929 945 961 977 993 1009 2 18 34 50 66 82 98 114 130 146 162 178 194 210 226 242 258 274 290 306 322 338 354 370 386 402 418 434 450 466 482 498 514 530 546 562 578 594 610 626 642 658 674 690 706 722 738 754 770 786 802 818 834 850 866 882 898 914 930 946 962 978 994 1010 3 19 35 51 67 83 99 115 131 147 163 179 195 211 227 243 259 275 291 307 323 339 355 371 387 403 419 435 451 467 483 499 515 531 547 563 579 595 611 627 643 659 675 691 707 723 739 755 771 787 803 819 835 851 867 883 899 915 931 947 963 979 995 1011 4 20 36 52 68 84 100 116 132 148 164 180 196 212 228 244 260 276 292 308 324 340 356 372 388 404 420 436 452 468 484 500 516 532 548 564 580 596 612 628 644 660 676 692 708 724 740 756 772 788 804 820 836 852 868 884 900 916 932 948 964 980 996 1012 5 21 37 53 69 85 101 117 133 149 165 181 197 213 229 245 261 277 293 309 325 341 357 373 389 405 421 437 453 469 485 501 517 533 549 565 581 597 613 629 645 661 677 693 709 725 741 757 773 789 805 821 837 853 869 885 901 917 933 949 965 981 997 1013 6 22 38 54 70 86 102 118 134 150 166 182 198 214 230 246 262 278 294 310 326 342 358 374 390 406 422 438 454 470 486 502 518 534 550 566 582 598 614 630 646 662 678 694 710 726 742 758 774 790 806 822 838 854 870 886 902 918 934 950 966 982 998 1014 7 23 39 55 71 87 103 119 135 151 167 183 199 215 231 247 263 279 295 311 327 343 359 375 391 407 423 439 455 471 487 503 519 535 551 567 583 599 615 631 647 663 679 695 711 727 743 759 775 791 807 823 839 855 871 887 903 919 935 951 967 983 999 1015 8 24 40 56 72 88 104 120 136 152 168 184 200 216 232 248 264 280 296 312 328 344 360 376 392 408 424 440 456 472 488 504 520 536 552 568 584 600 616 632 648 664 680 696 712 728 744 760 776 792 808 824 840 856 872 888 904 920 936 952 968 984 1000 1016 9 25 41 57 73 89 105 121 137 153 169 185 201 217 233 249 265 281 297 313 329 345 361 377 393 409 425 441 457 473 489 505 521 537 553 569 585 601 617 633 649 665 681 697 713 729 745 761 777 793 809 825 841 857 873 889 905 921 937 953 969 985 1001 1017 10 26 42 58 74 90 106 122 138 154 170 186 202 218 234 250 266 282 298 314 330 346 362 378 394 410 426 442 458 474 490 506 522 538 554 570 586 602 618 634 650 666 682 698 714 730 746 762 778 794 810 826 842 858 874 890 906 922 938 954 970 986 1002 1018 11 27 43 59 75 91 107 123 139 155 171 187 203 219 235 251 267 283 299 315 331 347 363 379 395 411 427 443 459 475 491 507 523 539 555 571 587 603 619 635 651 667 683 699 715 731 747 763 779 795 811 827 843 859 875 891 907 923 939 955 971 987 1003 1019 12 28 44 60 76 92 108 124 140 156 172 188 204 220 236 252 268 284 300 316 332 348 364 380 396 412 428 444 460 476 492 508 524 540 556 572 588 604 620 636 652 668 684 700 716 732 748 764 780 796 812 828 844 860 876 892 908 924 940 956 972 988 1004 1020 13 29 45 61 77 93 109 125 141 157 173 189 205 221 237 253 269 285 301 317 333 349 365 381 397 413 429 445 461 477 493 509 525 541 557 573 589 605 621 637 653 669 685 701 717 733 749 765 781 797 813 829 845 861 877 893 909 925 941 957 973 989 1005 1021 14 30 46 62 78 94 110 126 142 158 174 190 206 222 238 254 270 286 302 318 334 350 366 382 398 414 430 446 462 478 494 510 526 542 558 574 590 606 622 638 654 670 686 702 718 734 750 766 782 798 814 830 846 862 878 894 910 926 942 958 974 990 1006 1022 15 31 47 63 79 95 111 127 143 159 175 191 207 223 239 255 271 287 303 319 335 351 367 383 399 415 431 447 463 479 495 511 527 543 559 575 591 607 623 639 655 671 687 703 719 735 751 767 783 799 815 831 847 863 879 895 911 927 943 959 975 991 1007 1023]  arith_type=Unsigned  n_bits=10  bin_pt=0  latency=1  init_zero=on  explicit_period=off  period=1  rst=off  init_reg=0  en=off  dbl_ovrd=off  show_param=off  distributed_mem=on  use_rpm=off  gen_core=off
      settings: xl_area=[0, 0, 0, 0, 0, 0, 0]
  post_sync_delay : xbsIndex_r3/Delay  latency=4  reg_retiming=off  explicit_period=off  period=1  en=off  accept_only_valid=off  init_zero=on  dbl_ovrd=off  show_param=off
      settings: xl_area=[0, 0, 0, 0, 0, 0, 0]
  pre_sync_delay : xbsIndex_r3/Delay  latency=1  reg_retiming=off  explicit_period=off  period=1  en=off  accept_only_valid=off  init_zero=on  dbl_ovrd=off  show_param=off
      settings: xl_area=[0, 0, 0, 0, 0, 0, 0]
  sync_delay_en : casper_library/Delays/sync_delay_en  DelayLen=1024
      link override Constant: equ=P=C
      link override Constant1: equ=P=C
      link override Constant2: equ=P=C
      link override Constant3: equ=P=C
  sync_out : Outport
  valid : Outport  Port=2
  dout0 : Outport  Port=3
  wires:
  sync/1 -> Counter/1, pre_sync_delay/1
  en/1 -> Counter/2, sync_delay_en/2, delay_we/1
  Counter/1 -> Slice1/1, Slice2/1
  Slice1/1 -> delay_sel/1
  Slice2/1 -> delay_d0/1, map1/1
  pre_sync_delay/1 -> sync_delay_en/1
  sync_delay_en/1 -> post_sync_delay/1
  post_sync_delay/1 -> sync_out/1
  delay_we/1 -> delay_valid/1, dbl_buffer0/5
  delay_valid/1 -> valid/1
  delay_d0/1 -> dbl_buffer0/2
  map1/1 -> dbl_buffer0/3
  delay_sel/1 -> dbl_buffer0/1
  din0/1 -> delay_din0/1
  delay_din0/1 -> dbl_buffer0/4
  dbl_buffer0/1 -> dout0/1

== system pasp_16ip_16ch/pasp/fft_wideband_real/fft_biplex_real_4x0 ==
  pol1 : Inport  Port=1  LatchInput=off
  pol2 : Inport  Port=2  LatchInput=off
  pol3 : Inport  Port=3  LatchInput=off
  pol4 : Inport  Port=4  LatchInput=off
  sync : Inport  Port=5  LatchInput=off
  shift : Inport  Port=6  LatchInput=off
  bi_real_unscr_4x : Subsystem  mask{FFTSize=3, bram_latency=2}
      mask prompts: FFTSize "Size of FFT (2^?):"; bram_latency "BRAM Latency"
      mask init:
      | blk = gcb;
      | 
      | set_param([blk,'/reorder'],'map', mat2str(bit_reverse(0:2^(FFTSize-1)-1, FFTSize-1)));
      | set_param([blk,'/reorder'],'bram_latency', num2str(bram_latency));
      | set_param([blk,'/reorder1'],'map', mat2str(bit_reverse(2^(FFTSize-1)-1:-1:0, FFTSize-1)));
      | set_param([blk,'/reorder1'],'bram_latency', num2str(bram_latency));
      | set_param([blk,'/reorder2'],'map', mat2str(2^(FFTSize-1)-1:-1:0));
      | set_param([blk,'/reorder2'],'bram_latency', num2str(bram_latency));
  biplex_core : Subsystem  AncestorBlock=casper_library/FFTs/biplex_core  mask(biplex_core){FFTSize=3, BitWidth=18, quantization=Truncate, overflow=Wrap, add_latency=2, mult_latency=3, bram_latency=2}
      mask prompts: FFTSize "Size of FFT: (2^? pnts)"; BitWidth "Bitwidth: (Max Efficiency at 18 bits)"; quantization "Quantization Behavior"; overflow "Overflow Behavior"; add_latency "Add Latency"; mult_latency "Mult Latency"; bram_latency "BRAM Latency"
      mask init:
      | biplex_core_init(gcb,...
      |     'FFTSize', FFTSize,...
      |     'BitWidth', BitWidth,...
      |     'quantization', quantization,...
      |     'overflow', overflow,...
      |     'add_latency', add_latency,...
      |     'mult_latency', mult_latency,...
      |     'bram_latency', bram_latency);
      settings: AttributesFormatString=FFTSize=3
      mask StyleString: edit,edit,popup(Truncate|Round  (unbiased: +/- Inf)|Round  (unbiased: Even Values)),popup(Wrap|Saturate|Error),edit,edit,edit
  ri_to_c : Subsystem
  ri_to_c1 : Subsystem
  pol1_out : Outport
  pol2_out : Outport  Port=2
  pol3_out : Outport  Port=3
  pol4_out : Outport  Port=4
  of : Outport  Port=5
  sync_out : Outport  Port=6
  wires:
  bi_real_unscr_4x/5(sync_out) -> sync_out/1
  bi_real_unscr_4x/4(pol4_out) -> pol4_out/1
  bi_real_unscr_4x/3(pol3_out) -> pol3_out/1
  bi_real_unscr_4x/2(pol2_out) -> pol2_out/1
  bi_real_unscr_4x/1(pol1_out) -> pol1_out/1
  shift/1 -> biplex_core/4(shift)
  sync/1 -> biplex_core/3(sync)
  pol4/1 -> ri_to_c1/2(im)
  ri_to_c1/1(c) -> biplex_core/2(pol2)
  pol3/1 -> ri_to_c1/1(re)
  pol2/1 -> ri_to_c/2(im)
  ri_to_c/1(c) -> biplex_core/1(pol1)
  pol1/1 -> ri_to_c/1(re)
  biplex_core/3(of) -> of/1
  biplex_core/1(out1) -> bi_real_unscr_4x/1(even)
  biplex_core/2(out2) -> bi_real_unscr_4x/2(odd)
  biplex_core/4(sync_out) -> bi_real_unscr_4x/3(sync)

== system pasp_16ip_16ch/pasp/fft_wideband_real/fft_direct ==
  sync : Inport  Port=1  LatchInput=off
  shift : Inport  Port=2  LatchInput=off
  in0 : Inport  Port=3  LatchInput=off
  in1 : Inport  Port=4  LatchInput=off
  in2 : Inport  Port=5  LatchInput=off
  in3 : Inport  Port=6  LatchInput=off
  butterfly1_0 : Subsystem  AncestorBlock=casper_library/FFTs/butterfly_direct  mask(butterfly_direct){FFTSize=5, Coeffs=[0 4 2 6 1 5 3 7], StepPeriod=0, BitWidth=18, add_latency=2, mult_latency=3, bram_latency=2, use_bram=1, quantization=Truncate, overflow=Wrap}
      mask prompts: FFTSize "Size of FFT: (2^?)"; Coeffs "Coefficients: (0 to 2^(FFTSize-1)-1)"; StepPeriod "Coefficient Step Period: (2^?)"; BitWidth "Output Bitwidth:"; add_latency "Add Latency"; mult_latency "Mult Latency"; bram_latency "BRAM Latency"; use_bram "Store Coefficients in BRAM"; quantization "Quantization Behavior"; overflow "Overflow Behavior"
      mask init:
      | butterfly_direct_init(gcb,...
      |               'FFTSize', FFTSize,...
      |               'Coeffs', Coeffs,...
      |               'StepPeriod', StepPeriod,...
      |               'BitWidth', BitWidth,...
      |               'add_latency', add_latency,...
      |               'mult_latency', mult_latency,...
      |               'bram_latency', bram_latency,...
      |               'use_bram',use_bram,...
      |               'quantization',quantization,...
      |               'overflow',overflow);
      settings: AttributesFormatString=|
      | FFTSize=5, Coeffs=[0  4  2  6  1  5  3  7],
      |  StepPeriod=0, BitWidth=18
      mask StyleString: edit,edit,edit,edit,edit,edit,edit,edit,popup(Truncate|Round  (unbiased: +/- Inf)|Round  (unbiased: Even Values)),popup(Wrap|Saturate|Error)
  butterfly1_1 : Subsystem  AncestorBlock=casper_library/FFTs/butterfly_direct  mask(butterfly_direct){FFTSize=5, Coeffs=[0 4 2 6 1 5 3 7], StepPeriod=0, BitWidth=18, add_latency=2, mult_latency=3, bram_latency=2, use_bram=1, quantization=Truncate, overflow=Wrap}
      mask prompts: FFTSize "Size of FFT: (2^?)"; Coeffs "Coefficients: (0 to 2^(FFTSize-1)-1)"; StepPeriod "Coefficient Step Period: (2^?)"; BitWidth "Output Bitwidth:"; add_latency "Add Latency"; mult_latency "Mult Latency"; bram_latency "BRAM Latency"; use_bram "Store Coefficients in BRAM"; quantization "Quantization Behavior"; overflow "Overflow Behavior"
      mask init: same as pasp_16ip_16ch/pasp/fft_wideband_real/fft_direct/butterfly1_0
      settings: AttributesFormatString=|
      | FFTSize=5, Coeffs=[0  4  2  6  1  5  3  7],
      |  StepPeriod=0, BitWidth=18
      mask StyleString: edit,edit,edit,edit,edit,edit,edit,edit,popup(Truncate|Round  (unbiased: +/- Inf)|Round  (unbiased: Even Values)),popup(Wrap|Saturate|Error)
  butterfly2_0 : Subsystem  AncestorBlock=casper_library/FFTs/butterfly_direct  mask(butterfly_direct){FFTSize=5, Coeffs=[0 8 4 12 2 10 6 14], StepPeriod=0, BitWidth=18, add_latency=2, mult_latency=3, bram_latency=2, use_bram=1, quantization=Truncate, overflow=Wrap}
      mask prompts: FFTSize "Size of FFT: (2^?)"; Coeffs "Coefficients: (0 to 2^(FFTSize-1)-1)"; StepPeriod "Coefficient Step Period: (2^?)"; BitWidth "Output Bitwidth:"; add_latency "Add Latency"; mult_latency "Mult Latency"; bram_latency "BRAM Latency"; use_bram "Store Coefficients in BRAM"; quantization "Quantization Behavior"; overflow "Overflow Behavior"
      mask init: same as pasp_16ip_16ch/pasp/fft_wideband_real/fft_direct/butterfly1_0
      settings: AttributesFormatString=|
      | FFTSize=5, Coeffs=[0   8   4  12   2  10   6  14],
      |  StepPeriod=0, BitWidth=18
      mask StyleString: edit,edit,edit,edit,edit,edit,edit,edit,popup(Truncate|Round  (unbiased: +/- Inf)|Round  (unbiased: Even Values)),popup(Wrap|Saturate|Error)
  butterfly2_1 : Subsystem  AncestorBlock=casper_library/FFTs/butterfly_direct  mask(butterfly_direct){FFTSize=5, Coeffs=[1 9 5 13 3 11 7 15], StepPeriod=0, BitWidth=18, add_latency=2, mult_latency=3, bram_latency=2, use_bram=1, quantization=Truncate, overflow=Wrap}
      mask prompts: FFTSize "Size of FFT: (2^?)"; Coeffs "Coefficients: (0 to 2^(FFTSize-1)-1)"; StepPeriod "Coefficient Step Period: (2^?)"; BitWidth "Output Bitwidth:"; add_latency "Add Latency"; mult_latency "Mult Latency"; bram_latency "BRAM Latency"; use_bram "Store Coefficients in BRAM"; quantization "Quantization Behavior"; overflow "Overflow Behavior"
      mask init: same as pasp_16ip_16ch/pasp/fft_wideband_real/fft_direct/butterfly1_0
      settings: AttributesFormatString=|
      | FFTSize=5, Coeffs=[1   9   5  13   3  11   7  15],
      |  StepPeriod=0, BitWidth=18
      mask StyleString: edit,edit,edit,edit,edit,edit,edit,edit,popup(Truncate|Round  (unbiased: +/- Inf)|Round  (unbiased: Even Values)),popup(Wrap|Saturate|Error)
  node0_{0..3} (4 alike) : xbsIndex_r3/Delay  latency=0  reg_retiming=off  explicit_period=off  period=1  en=off  accept_only_valid=off  init_zero=on  dbl_ovrd=off  show_param=off
      settings: xl_area=[0, 0, 0, 0, 0, 0, 0]
  node1_{0..3} (4 alike) : xbsIndex_r3/Delay  latency=0  reg_retiming=off  explicit_period=off  period=1  en=off  accept_only_valid=off  init_zero=on  dbl_ovrd=off  show_param=off
      settings: xl_area=[0, 0, 0, 0, 0, 0, 0]
  node2_{0..3} (4 alike) : xbsIndex_r3/Delay  latency=0  reg_retiming=off  explicit_period=off  period=1  en=off  accept_only_valid=off  init_zero=on  dbl_ovrd=off  show_param=off
      settings: xl_area=[0, 0, 0, 0, 0, 0, 0]
  slice0 : xbsIndex_r3/Slice  mode=Lower Bit Location + Width  nbits=1  bit1=0  base1=MSB of Input  bit0=0  base0=LSB of Input  boolean_output=on  explicit_period=off  period=1  dbl_ovrd=off
  slice1 : xbsIndex_r3/Slice  mode=Lower Bit Location + Width  nbits=1  bit1=0  base1=MSB of Input  bit0=1  base0=LSB of Input  boolean_output=on  explicit_period=off  period=1  dbl_ovrd=off
  sync_out : Outport
  out0 : Outport  Port=2
  out1 : Outport  Port=3
  out2 : Outport  Port=4
  out3 : Outport  Port=5
  wires:
  in0/1 -> node0_0/1
  in1/1 -> node0_1/1
  in2/1 -> node0_2/1
  in3/1 -> node0_3/1
  shift/1 -> slice0/1, slice1/1
  node2_0/1 -> out0/1
  node2_1/1 -> out2/1
  node2_2/1 -> out1/1
  node2_3/1 -> out3/1
  node0_0/1 -> butterfly1_0/1(a)
  node0_2/1 -> butterfly1_0/2(b)
  butterfly1_0/1(a+bw) -> node1_0/1
  butterfly1_0/2(a-bw) -> node1_2/1
  sync/1 -> butterfly1_0/3(sync), butterfly1_1/3(sync)
  slice0/1 -> butterfly1_0/4(shift), butterfly1_1/4(shift)
  node0_1/1 -> butterfly1_1/1(a)
  node0_3/1 -> butterfly1_1/2(b)
  butterfly1_1/1(a+bw) -> node1_1/1
  butterfly1_1/2(a-bw) -> node1_3/1
  node1_0/1 -> butterfly2_0/1(a)
  node1_1/1 -> butterfly2_0/2(b)
  butterfly2_0/1(a+bw) -> node2_0/1
  butterfly2_0/2(a-bw) -> node2_1/1
  butterfly1_0/4(sync_out) -> butterfly2_0/3(sync)
  butterfly2_0/4(sync_out) -> sync_out/1
  slice1/1 -> butterfly2_0/4(shift), butterfly2_1/4(shift)
  node1_2/1 -> butterfly2_1/1(a)
  node1_3/1 -> butterfly2_1/2(b)
  butterfly2_1/1(a+bw) -> node2_2/1
  butterfly2_1/2(a-bw) -> node2_3/1
  butterfly1_1/4(sync_out) -> butterfly2_1/3(sync)
